simulink model "testiranje_kontrolera_sim"  (R2020a)
settings: Solver=FixedStepAuto  StartTime=0.0  StopTime=sim_duration  FixedStep=1e-4  RelTol=1e-3
undefined symbols (not defined in the file): C, E, Kp, L, R, sim_duration, Td, Tf, Ti, Tt, ue, x2e
libraries: cstblocks x2
settings Model: Creator=HP  LastModifiedBy=HP

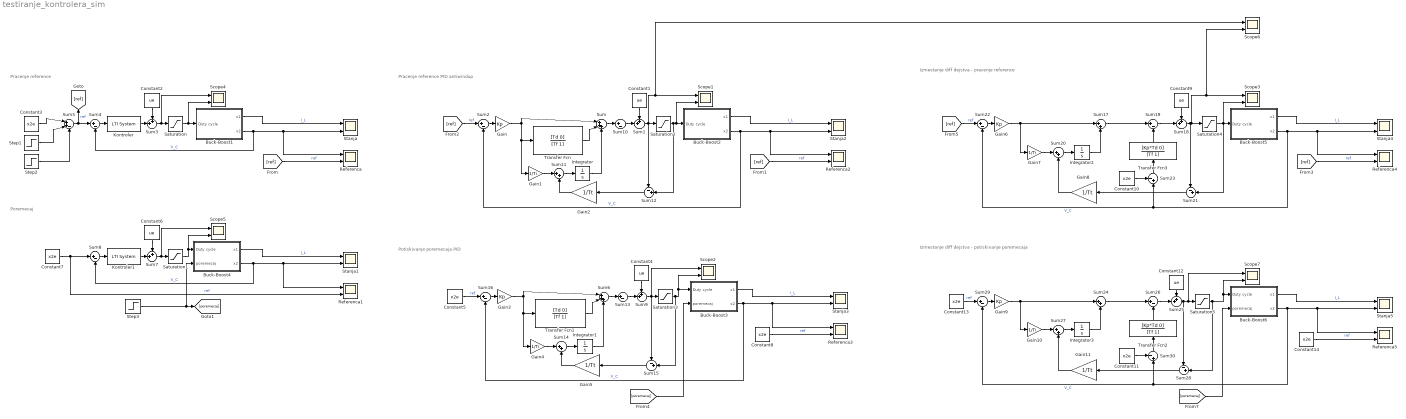
== system testiranje_kontrolera_sim ==
  note: Izmestanje diff dejstva - pracenje reference
  note: Pracenje reference
  note: Poremecaj
  note: Pracenje reference PID
      |
      | antiwindup
  note: Potiskivanje poremecaja PID
  note: Izmestanje diff dejstva - potiskivanje poremecaja
  Buck-Boost1 : Subsystem
  Buck-Boost2 : Subsystem
  Buck-Boost3 : Subsystem
  Buck-Boost4 : Subsystem
  Buck-Boost5 : Subsystem
  Buck-Boost6 : Subsystem
  Constant{1..2,4,6,9,12} (6 alike) : Constant  Value=ue
  Constant{3,5,7..8,10..11,13..14} (8 alike) : Constant  Value=x2e
  Gain{,3,6,9} (4 alike) : Gain  Gain=Kp
  Gain{1,4,7,10} (4 alike) : Gain  Gain=1/Ti
  Gain{2,5,8,11} (4 alike) : Gain  Gain=1/Tt
  Integrator{,1..3} (4 alike) : Integrator
  Kontroler : cstblocks/LTI System  sys=Kontroler  IC=[]
  Kontroler1 : cstblocks/LTI System  sys=Kontroler  IC=[]
  Referenca{,1..5} (6 alike) : Scope  NumInputPorts=2
  Saturation{,1..5} (6 alike) : Saturate  UpperLimit=1  LowerLimit=0
  Scope{1..7} (7 alike) : Scope  NumInputPorts=2
  Stanja{,1..5} (6 alike) : Scope  NumInputPorts=2
  Step1 : Step  Time=0.3*sim_duration  After=0.05 * x2e  SampleTime=0
  Step2 : Step  Time=0.7*sim_duration  After=0.1* x2e  SampleTime=0
  Step3 : Step  Time=0.5*sim_duration  After=0.1*E  SampleTime=0
  Sum : Sum  Inputs=|+++
  Sum{1,3,7,9,18,25} (6 alike) : Sum  Inputs=++|
  Sum{2,4,8,10,13,16,19,22,26,29} (10 alike) : Sum  Inputs=|+-
  Sum{11,14,17,20,24,27} (6 alike) : Sum  Inputs=|++
  Sum{12,15,21,23,28,30} (6 alike) : Sum  Inputs=-+|
  Sum5 : Sum  Inputs=|++-
  Sum6 : Sum  Inputs=|+++
  Transfer Fcn : TransferFcn  Numerator=[Td 0]  Denominator=[Tf 1]
  Transfer Fcn1 : TransferFcn  Numerator=[Td 0]  Denominator=[Tf 1]
  Transfer Fcn2 : TransferFcn  Numerator=[Kp*Td 0]  Denominator=[Tf 1]
  Transfer Fcn3 : TransferFcn  Numerator=[Kp*Td 0]  Denominator=[Tf 1]
  wires:
  Sum3/1 -> Scope4/1, Saturation/1
  Constant2/1 -> Sum3/1
  Buck-Boost1/2(x2) -> Referenca/1, Stanja/2, Sum4/2  "V_C"
  Buck-Boost1/1(x1) -> Stanja/1  "I_L"
  Constant3/1 -> Sum5/1
  Sum5/1 -> Sum4/1, [ref]  "ref"
  Step1/1 -> Sum5/2
  Step2/1 -> Sum5/3
  Saturation/1 -> Scope4/2, Buck-Boost1/1(Duty cycle)
  [ref] -> Referenca/2  "ref"
  Kontroler1/1 -> Sum7/2
  Buck-Boost4/1(x1) -> Stanja1/1  "I_L"
  Saturation1/1 -> Scope5/2, Buck-Boost4/1(Duty cycle)
  Constant6/1 -> Sum7/1
  Constant7/1 -> Referenca1/2, Sum8/1  "ref"
  Buck-Boost4/2(x2) -> Referenca1/1, Stanja1/2, Sum8/2  "V_C"
  Sum7/1 -> Scope5/1, Saturation1/1
  Step3/1 -> [poremecaj], Buck-Boost4/2(poremecaj)
  Kontroler/1 -> Sum3/2
  Sum4/1 -> Kontroler/1
  Sum8/1 -> Kontroler1/1
  Sum10/1 -> Sum1/2
  Sum1/1 -> Sum12/1, Scope6/1, Scope1/1, Saturation2/1
  [ref] -> Referenca2/2  "ref"
  Sum2/1 -> Gain/1
  Buck-Boost2/1(x1) -> Stanja2/1  "I_L"
  [ref] -> Sum2/1  "ref"
  Constant1/1 -> Sum1/1
  Buck-Boost2/2(x2) -> Referenca2/1, Stanja2/2, Sum2/2  "V_C"
  Sum/1 -> Sum10/1
  Gain1/1 -> Sum11/1
  Sum11/1 -> Integrator/1
  Gain2/1 -> Sum11/2
  Sum12/1 -> Gain2/1
  Saturation2/1 -> Sum12/2, Scope1/2, Buck-Boost2/1(Duty cycle)
  Transfer Fcn/1 -> Sum/2
  Gain/1 -> Sum/1, Transfer Fcn/1, Gain1/1
  Integrator/1 -> Sum/3
  Transfer Fcn1/1 -> Sum6/2
  Sum6/1 -> Sum13/1
  Sum14/1 -> Integrator1/1
  Gain4/1 -> Sum14/1
  Sum16/1 -> Gain3/1
  Integrator1/1 -> Sum6/3
  Gain5/1 -> Sum14/2
  Buck-Boost3/2(x2) -> Referenca3/1, Stanja3/2, Sum16/2  "V_C"
  Buck-Boost3/1(x1) -> Stanja3/1  "I_L"
  Constant8/1 -> Referenca3/2  "ref"
  Constant5/1 -> Sum16/1  "ref"
  Sum13/1 -> Sum9/2
  Saturation3/1 -> Sum15/2, Buck-Boost3/1(Duty cycle), Scope2/2
  Sum15/1 -> Gain5/1
  Gain3/1 -> Sum6/1, Transfer Fcn1/1, Gain4/1
  Constant4/1 -> Sum9/1
  Sum9/1 -> Sum15/1, Scope2/1, Saturation3/1
  [poremecaj] -> Buck-Boost3/2(poremecaj)
  Gain7/1 -> Sum20/1
  Sum20/1 -> Integrator2/1
  Sum17/1 -> Sum19/1
  Integrator2/1 -> Sum17/2
  Constant9/1 -> Sum18/1
  [ref] -> Sum22/1  "ref"
  Buck-Boost5/1(x1) -> Stanja4/1  "I_L"
  [ref] -> Referenca4/2  "ref"
  Saturation4/1 -> Buck-Boost5/1(Duty cycle), Sum21/2, Scope3/2
  Sum21/1 -> Gain8/1
  Gain8/1 -> Sum20/2
  Gain6/1 -> Sum17/1, Gain7/1
  Sum22/1 -> Gain6/1
  Buck-Boost5/2(x2) -> Referenca4/1, Stanja4/2, Sum22/2, Sum23/2  "V_C"
  Sum19/1 -> Sum18/2
  Sum18/1 -> Saturation4/1, Scope6/2, Scope3/1, Sum21/1
  Transfer Fcn3/1 -> Sum19/2
  Sum23/1 -> Transfer Fcn3/1
  Constant10/1 -> Sum23/1
  Sum30/1 -> Transfer Fcn2/1
  Transfer Fcn2/1 -> Sum26/2
  Buck-Boost6/1(x1) -> Stanja5/1  "I_L"
  Sum29/1 -> Gain9/1
  Buck-Boost6/2(x2) -> Referenca5/1, Stanja5/2, Sum29/2, Sum30/2  "V_C"
  Sum25/1 -> Scope7/1, Saturation5/1, Sum28/1
  Gain11/1 -> Sum27/2
  Constant12/1 -> Sum25/1
  Gain9/1 -> Sum24/1, Gain10/1
  Sum24/1 -> Sum26/1
  Constant14/1 -> Referenca5/2  "ref"
  Integrator3/1 -> Sum24/2
  Constant11/1 -> Sum30/1
  Sum26/1 -> Sum25/2
  Sum27/1 -> Integrator3/1
  Gain10/1 -> Sum27/1
  Sum28/1 -> Gain11/1
  Saturation5/1 -> Buck-Boost6/1(Duty cycle), Scope7/2, Sum28/2
  Constant13/1 -> Sum29/1  "ref"
  [poremecaj] -> Buck-Boost6/2(poremecaj)

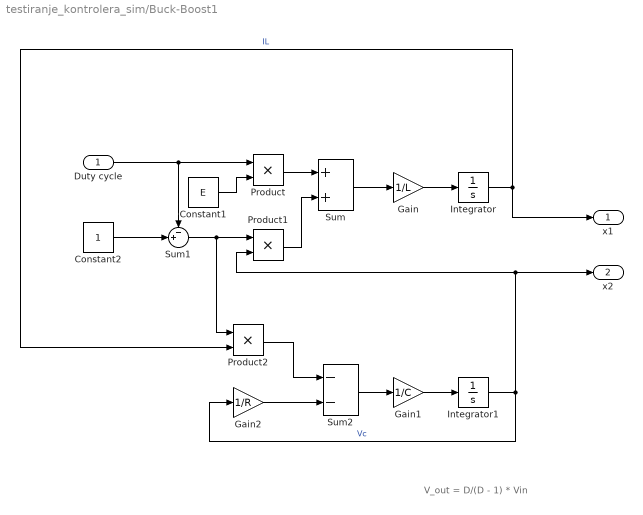
== system testiranje_kontrolera_sim/Buck-Boost1 ==
  note: V_out = D/(D - 1) * Vin
  Duty cycle : Inport
  Constant1 : Constant  Value=E
  Constant2 : Constant
  Gain : Gain  Gain=1/L
  Gain1 : Gain  Gain=1/C
  Gain2 : Gain  Gain=1/R
  Integrator : Integrator
  Integrator1 : Integrator
  Product : Product
  Product1 : Product
  Product2 : Product
  Sum : Sum
  Sum1 : Sum  Inputs=-+|
  Sum2 : Sum  Inputs=--
  x1 : Outport
  x2 : Outport  Port=2
  wires:
  Product/1 -> Sum/1
  Product1/1 -> Sum/2
  Sum2/1 -> Gain1/1
  Constant1/1 -> Product/2
  Integrator1/1 -> Gain2/1, x2/1, Product1/2  "Vc"
  Gain1/1 -> Integrator1/1
  Constant2/1 -> Sum1/2
  Integrator/1 -> x1/1, Product2/2  "IL"
  Sum/1 -> Gain/1
  Gain2/1 -> Sum2/2
  Sum1/1 -> Product2/1, Product1/1
  Duty cycle/1 -> Sum1/1, Product/1
  Product2/1 -> Sum2/1
  Gain/1 -> Integrator/1

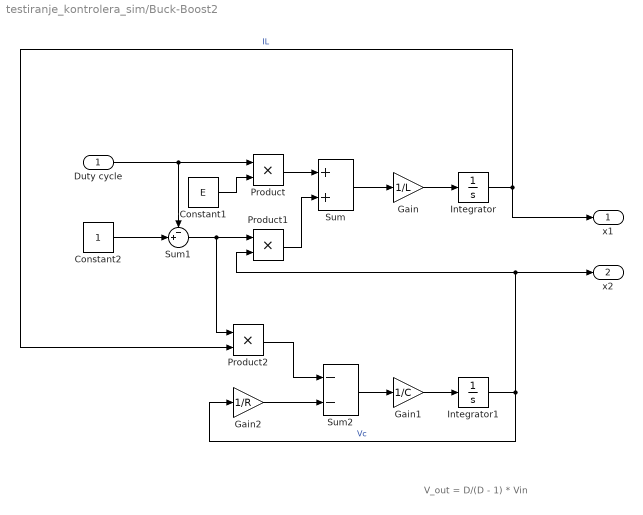
== system testiranje_kontrolera_sim/Buck-Boost2 ==
  note: V_out = D/(D - 1) * Vin
  Duty cycle : Inport
  Constant1 : Constant  Value=E
  Constant2 : Constant
  Gain : Gain  Gain=1/L
  Gain1 : Gain  Gain=1/C
  Gain2 : Gain  Gain=1/R
  Integrator : Integrator
  Integrator1 : Integrator
  Product : Product
  Product1 : Product
  Product2 : Product
  Sum : Sum
  Sum1 : Sum  Inputs=-+|
  Sum2 : Sum  Inputs=--
  x1 : Outport
  x2 : Outport  Port=2
  wires:
  Product/1 -> Sum/1
  Product1/1 -> Sum/2
  Sum2/1 -> Gain1/1
  Constant1/1 -> Product/2
  Integrator1/1 -> Gain2/1, x2/1, Product1/2  "Vc"
  Gain1/1 -> Integrator1/1
  Constant2/1 -> Sum1/2
  Integrator/1 -> x1/1, Product2/2  "IL"
  Sum/1 -> Gain/1
  Gain2/1 -> Sum2/2
  Sum1/1 -> Product2/1, Product1/1
  Duty cycle/1 -> Sum1/1, Product/1
  Product2/1 -> Sum2/1
  Gain/1 -> Integrator/1

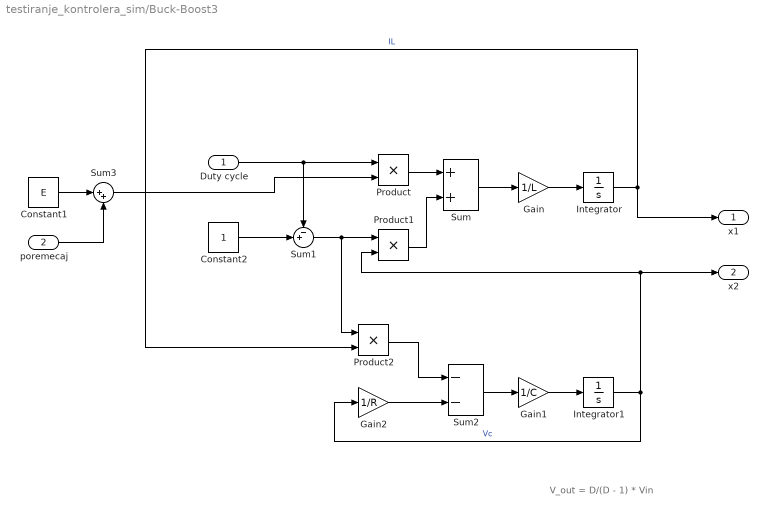
== system testiranje_kontrolera_sim/Buck-Boost3 ==
  note: V_out = D/(D - 1) * Vin
  Duty cycle : Inport
  poremecaj : Inport  Port=2
  Constant1 : Constant  Value=E
  Constant2 : Constant
  Gain : Gain  Gain=1/L
  Gain1 : Gain  Gain=1/C
  Gain2 : Gain  Gain=1/R
  Integrator : Integrator
  Integrator1 : Integrator
  Product : Product
  Product1 : Product
  Product2 : Product
  Sum : Sum
  Sum1 : Sum  Inputs=-+|
  Sum2 : Sum  Inputs=--
  Sum3 : Sum  Inputs=|++
  x1 : Outport
  x2 : Outport  Port=2
  wires:
  Product/1 -> Sum/1
  Product1/1 -> Sum/2
  Sum2/1 -> Gain1/1
  Integrator1/1 -> Gain2/1, x2/1, Product1/2  "Vc"
  Gain1/1 -> Integrator1/1
  Constant2/1 -> Sum1/2
  Integrator/1 -> x1/1, Product2/2  "IL"
  Sum/1 -> Gain/1
  Gain2/1 -> Sum2/2
  Sum1/1 -> Product2/1, Product1/1
  Duty cycle/1 -> Sum1/1, Product/1
  Product2/1 -> Sum2/1
  Gain/1 -> Integrator/1
  Constant1/1 -> Sum3/1
  Sum3/1 -> Product/2
  poremecaj/1 -> Sum3/2

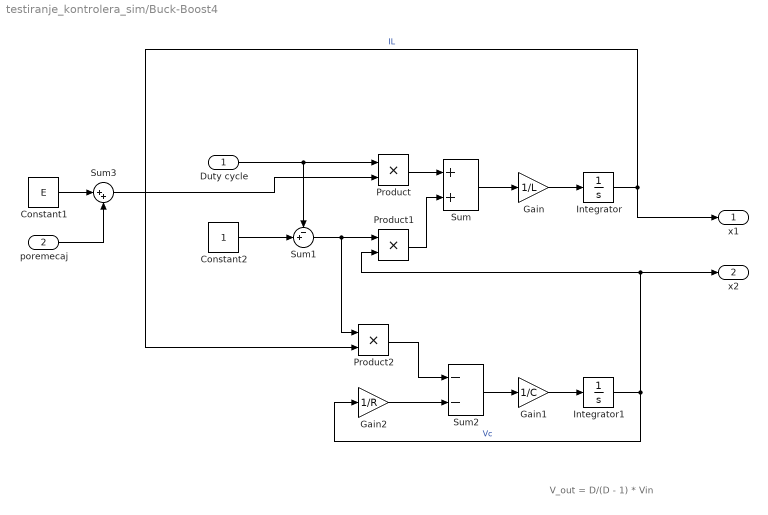
== system testiranje_kontrolera_sim/Buck-Boost4 ==
  note: V_out = D/(D - 1) * Vin
  Duty cycle : Inport
  poremecaj : Inport  Port=2
  Constant1 : Constant  Value=E
  Constant2 : Constant
  Gain : Gain  Gain=1/L
  Gain1 : Gain  Gain=1/C
  Gain2 : Gain  Gain=1/R
  Integrator : Integrator
  Integrator1 : Integrator
  Product : Product
  Product1 : Product
  Product2 : Product
  Sum : Sum
  Sum1 : Sum  Inputs=-+|
  Sum2 : Sum  Inputs=--
  Sum3 : Sum  Inputs=|++
  x1 : Outport
  x2 : Outport  Port=2
  wires:
  Product/1 -> Sum/1
  Product1/1 -> Sum/2
  Sum2/1 -> Gain1/1
  Integrator1/1 -> Gain2/1, x2/1, Product1/2  "Vc"
  Gain1/1 -> Integrator1/1
  Constant2/1 -> Sum1/2
  Integrator/1 -> x1/1, Product2/2  "IL"
  Sum/1 -> Gain/1
  Gain2/1 -> Sum2/2
  Sum1/1 -> Product2/1, Product1/1
  Duty cycle/1 -> Sum1/1, Product/1
  Product2/1 -> Sum2/1
  Gain/1 -> Integrator/1
  Constant1/1 -> Sum3/1
  Sum3/1 -> Product/2
  poremecaj/1 -> Sum3/2

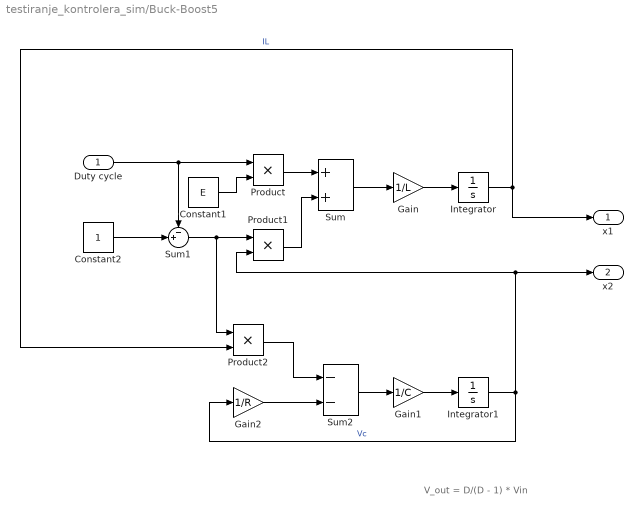
== system testiranje_kontrolera_sim/Buck-Boost5 ==
  note: V_out = D/(D - 1) * Vin
  Duty cycle : Inport
  Constant1 : Constant  Value=E
  Constant2 : Constant
  Gain : Gain  Gain=1/L
  Gain1 : Gain  Gain=1/C
  Gain2 : Gain  Gain=1/R
  Integrator : Integrator
  Integrator1 : Integrator
  Product : Product
  Product1 : Product
  Product2 : Product
  Sum : Sum
  Sum1 : Sum  Inputs=-+|
  Sum2 : Sum  Inputs=--
  x1 : Outport
  x2 : Outport  Port=2
  wires:
  Product/1 -> Sum/1
  Product1/1 -> Sum/2
  Sum2/1 -> Gain1/1
  Constant1/1 -> Product/2
  Integrator1/1 -> Gain2/1, x2/1, Product1/2  "Vc"
  Gain1/1 -> Integrator1/1
  Constant2/1 -> Sum1/2
  Integrator/1 -> x1/1, Product2/2  "IL"
  Sum/1 -> Gain/1
  Gain2/1 -> Sum2/2
  Sum1/1 -> Product2/1, Product1/1
  Duty cycle/1 -> Sum1/1, Product/1
  Product2/1 -> Sum2/1
  Gain/1 -> Integrator/1

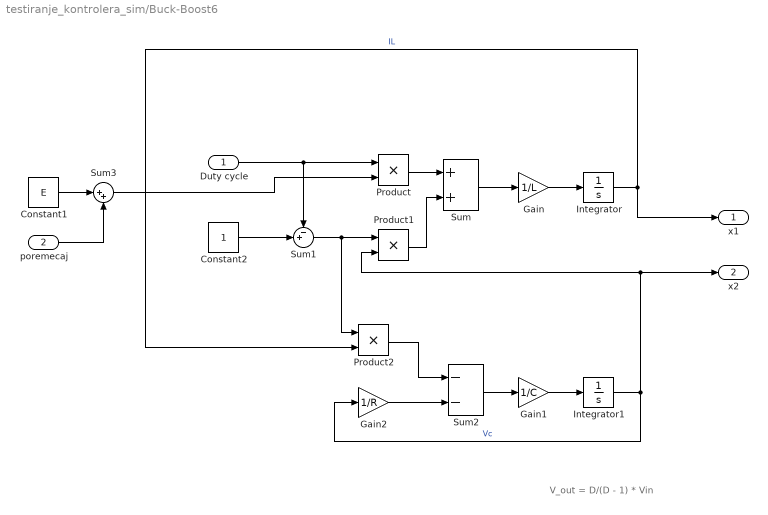
== system testiranje_kontrolera_sim/Buck-Boost6 ==
  note: V_out = D/(D - 1) * Vin
  Duty cycle : Inport
  poremecaj : Inport  Port=2
  Constant1 : Constant  Value=E
  Constant2 : Constant
  Gain : Gain  Gain=1/L
  Gain1 : Gain  Gain=1/C
  Gain2 : Gain  Gain=1/R
  Integrator : Integrator
  Integrator1 : Integrator
  Product : Product
  Product1 : Product
  Product2 : Product
  Sum : Sum
  Sum1 : Sum  Inputs=-+|
  Sum2 : Sum  Inputs=--
  Sum3 : Sum  Inputs=|++
  x1 : Outport
  x2 : Outport  Port=2
  wires:
  Product/1 -> Sum/1
  Product1/1 -> Sum/2
  Sum2/1 -> Gain1/1
  Integrator1/1 -> Gain2/1, x2/1, Product1/2  "Vc"
  Gain1/1 -> Integrator1/1
  Constant2/1 -> Sum1/2
  Integrator/1 -> x1/1, Product2/2  "IL"
  Sum/1 -> Gain/1
  Gain2/1 -> Sum2/2
  Sum1/1 -> Product2/1, Product1/1
  Duty cycle/1 -> Sum1/1, Product/1
  Product2/1 -> Sum2/1
  Gain/1 -> Integrator/1
  Constant1/1 -> Sum3/1
  Sum3/1 -> Product/2
  poremecaj/1 -> Sum3/2
